simulink model "ScriptDemo"  (R2022b)
settings: configuration reference "TmVcThermal_Configuration_sub" (kept outside this file)
undefined symbols (not defined in the file or in its folder): aaaa, bbbb, cTmComprCtrl_D_u8HvacFlowTable_db, cTmComprCtrl_D_u8HvacFlowTable_sw, cTmComprCtrl_n_i16ChillCmpIMax, cTmComprCtrl_n_i16ChillCmpIMin, cTmComprCtrl_n_i16ChillCmpIMin666, cTmComprCtrl_n_i16ChillCmpPMax, cTmComprCtrl_n_i16ChillCmpPMin, cTmComprCtrl_n_i16CmpChillCoolRpmKiMax, cTmComprCtrl_n_i16CmpChillCoolRpmKiMin, cTmComprCtrl_n_i16CmpChillCoolRpmKpMax, cTmComprCtrl_n_i16CmpChillCoolRpmKpMin, cTmComprCtrl_n_i16CmpCoolRpmKiMax, cTmComprCtrl_n_i16CmpCoolRpmKiMin, cTmComprCtrl_n_i16CmpCoolRpmKpMax, cTmComprCtrl_n_i16CmpCoolRpmKpMin, cTmComprCtrl_n_i16SM4CmpHeatKiMax, cTmComprCtrl_n_i16SM4CmpHeatKiMin, cTmComprCtrl_n_i16SM4CmpHeatKpMax, cTmComprCtrl_n_i16SM4CmpHeatKpMin, cTmComprCtrl_n_i16SM5CmpHeatKiMax, cTmComprCtrl_n_i16SM5CmpHeatKiMin, cTmComprCtrl_n_i16SM5CmpHeatKpMax, cTmComprCtrl_n_i16SM5CmpHeatKpMin, cTmComprCtrl_n_i16SM6CmpHeatKiMax, cTmComprCtrl_n_i16SM6CmpHeatKiMin, cTmComprCtrl_n_i16SM6CmpHeatKpMax, cTmComprCtrl_n_i16SM6CmpHeatKpMin, cTmComprCtrl_n_u16CmpMaxSpdFanFltLimt, cTmComprCtrl_n_u16CmpMaxSpdLoSidePFltLimt, cTmComprCtrl_n_u16CmpMaxSpdSensorFltLimt, cTmComprCtrl_n_u16CompMinRpm, cTmComprCtrl_n_u16CompRpmIncThres, cTmComprCtrl_t_u16BattCooltFFPeriod, cTmComprCtrl_t_u16BattCooltPIPeriod, cTmComprCtrl_t_u16CmpCoolFFPeriod, cTmComprCtrl_t_u16CmpCoolPIPeriod, cTmComprCtrl_t_u16CoolCmpChillFFPeriod, cTmComprCtrl_t_u16CoolCmpChillPIPeriod, cTmComprCtrl_t_u16SM4CmpHeatFFPeriod, cTmComprCtrl_t_u16SM4CmpHeatPIPeriod, cTmComprCtrl_t_u16SM5CmpHeatFFPeriod, cTmComprCtrl_t_u16SM5CmpHeatPIPeriod, cTmComprCtrl_t_u16SM6CmpHeatFFPeriod, cTmComprCtrl_t_u16SM6CmpHeatPIPeriod, cTmComprCtrl_Te_EvapClearInteg, cTmComprCtrl_Te_i16HpReqTempSaturoffset, cTmComprCtrl_Te_i16SatLpReplaceDiff, cTmComprCtrl_Te_i16SM3BatDiffStartEvapDecOffset, cTmComprCtrl_Te_i16SM3EvapLo, cTmComprCtrl_Te_i16SM3TBatDiffEntEvapDecOffset, cTmComprCtrl_Te_i16SM3TBatDiffEntEvapDecOffsetQuit, cTmComprCtrl_Te_s32ErrCmpChillPIContinueCoolH, cTmComprCtrl_Te_s32ErrCmpChillPIContinueCoolL, cTmComprCtrl_Te_s32ErrCmpPIContinueChillH, cTmComprCtrl_Te_s32ErrCmpPIContinueChillL, cTmComprCtrl_Te_s32ErrCmpPIContinueCoolH, cTmComprCtrl_Te_s32ErrCmpPIContinueCoolL, cTmComprCtrl_Te_s32ErrCmpPIContinueHeatH ... (+398)
libraries: simulink x846, PCMULib x711, simulink_need_slupdate x4
(part 25 of 49)

== system ScriptDemo/Create/createSigOnLine/Before2/Before ==
  note: % 目的: 为输出端口创建debug 及对应的输入模块
      | [cnt] = createDebug(gcs)
  sTmRefriVlvCtrl_X_s32CEXVPosReqIn : Inport  OutDataTypeStr=single
  sTmRefriVlvCtrl_X_s32EEXVPosReqIn : Inport  Port=2  OutDataTypeStr=single
  sTmRefriVlvCtrl_X_s32BEXVPosReqIn : Inport  Port=3  OutDataTypeStr=single
  yTmRefriVlvCtrl_B_HpcCexvMovEnableIn : Inport  Port=4  OutDataTypeStr=boolean
  sTmRefriVlvCtrl_Z_u8CEXVInitStateIn : Inport  Port=5  OutDataTypeStr=uint8
  yTmRefriVlvCtrl_B_CexvCalibReqIn : Inport  Port=6  OutDataTypeStr=boolean
  yTmRefriVlvCtrl_B_HpcEexvMovEnableIn : Inport  Port=7  OutDataTypeStr=boolean
  sTmRefriVlvCtrl_Z_u8EEXVInitStateIn : Inport  Port=8  OutDataTypeStr=uint8
  yTmRefriVlvCtrl_B_EexvCalibReqIn : Inport  Port=9  OutDataTypeStr=boolean
  yTmRefriVlvCtrl_B_HpcBexvMovEnableIn : Inport  Port=10  OutDataTypeStr=boolean
  sTmRefriVlvCtrl_Z_u8BEXVInitStateIn : Inport  Port=11  OutDataTypeStr=uint8
  yTmRefriVlvCtrl_B_BexvCalibReqIn : Inport  Port=12  OutDataTypeStr=boolean
  sTmRefriVlvCtrl_X_s32SM3BexvMaxPosIn : Inport  Port=13  OutDataTypeStr=single
  yTmRefriVlvCtrl_B_EvapBattTLimBexvEnaIn : Inport  Port=14  OutDataTypeStr=boolean
  sTmRefriVlvCtrl_D_u8EexvRefriSwitchStIn : Inport  Port=15  OutDataTypeStr=uint8
  sTmRefriVlvCtrl_D_u8CexvRefriSwitchStIn : Inport  Port=16  OutDataTypeStr=uint8
  sTmRefriVlvCtrl_D_u8BexvRefriSwitchStIn : Inport  Port=17  OutDataTypeStr=uint8
  OutDebug : PCMULib/Interface/OutdebugRvs  SWI=cTmRefriVlvCtrl_X_s32CEXVPosReq_sw  DBI=cTmRefriVlvCtrl_X_s32CEXVPosReq_db
      settings: SourceProductName=PCMULib
  OutDebug1 : PCMULib/Interface/OutdebugRvs  SWI=cTmRefriVlvCtrl_X_s32EEXVPosReq_sw  DBI=cTmRefriVlvCtrl_X_s32EEXVPosReq_db
      settings: SourceProductName=PCMULib
  OutDebug10 : PCMULib/Interface/OutdebugRvs  SWI=cTmRefriVlvCtrl_Z_u8BEXVInitState_sw  DBI=cTmRefriVlvCtrl_Z_u8BEXVInitState_db
      settings: SourceProductName=PCMULib
  OutDebug11 : PCMULib/Interface/OutdebugRvs  SWI=cTmRefriVlvCtrl_B_BexvCalibReq_sw  DBI=cTmRefriVlvCtrl_B_BexvCalibReq_db
      settings: SourceProductName=PCMULib
  OutDebug12 : PCMULib/Interface/OutdebugRvs  SWI=cTmRefriVlvCtrl_X_s32SM3BexvMaxPos_sw  DBI=cTmRefriVlvCtrl_X_s32SM3BexvMaxPos_db
      settings: SourceProductName=PCMULib
  OutDebug13 : PCMULib/Interface/OutdebugRvs  SWI=cTmRefriVlvCtrl_B_EvapBattTLimBexvEna_sw  DBI=cTmRefriVlvCtrl_B_EvapBattTLimBexvEna_db
      settings: SourceProductName=PCMULib
  OutDebug14 : PCMULib/Interface/OutdebugRvs  SWI=cTmRefriVlvCtrl_D_u8EexvRefriSwitchSt_sw  DBI=cTmRefriVlvCtrl_D_u8EexvRefriSwitchSt_db
      settings: SourceProductName=PCMULib
  OutDebug15 : PCMULib/Interface/OutdebugRvs  SWI=cTmRefriVlvCtrl_D_u8CexvRefriSwitchSt_sw  DBI=cTmRefriVlvCtrl_D_u8CexvRefriSwitchSt_db
      settings: SourceProductName=PCMULib
  OutDebug16 : PCMULib/Interface/OutdebugRvs  SWI=cTmRefriVlvCtrl_D_u8BexvRefriSwitchSt_sw  DBI=cTmRefriVlvCtrl_D_u8BexvRefriSwitchSt_db
      settings: SourceProductName=PCMULib
  OutDebug2 : PCMULib/Interface/OutdebugRvs  SWI=cTmRefriVlvCtrl_X_s32BEXVPosReq_sw  DBI=cTmRefriVlvCtrl_X_s32BEXVPosReq_db
      settings: SourceProductName=PCMULib
  OutDebug3 : PCMULib/Interface/OutdebugRvs  SWI=cTmRefriVlvCtrl_B_HpcCexvMovEnable_sw  DBI=cTmRefriVlvCtrl_B_HpcCexvMovEnable_db
      settings: SourceProductName=PCMULib
  OutDebug4 : PCMULib/Interface/OutdebugRvs  SWI=cTmRefriVlvCtrl_Z_u8CEXVInitState_sw  DBI=cTmRefriVlvCtrl_Z_u8CEXVInitState_db
      settings: SourceProductName=PCMULib
  OutDebug5 : PCMULib/Interface/OutdebugRvs  SWI=cTmRefriVlvCtrl_B_CexvCalibReq_sw  DBI=cTmRefriVlvCtrl_B_CexvCalibReq_db
      settings: SourceProductName=PCMULib
  OutDebug6 : PCMULib/Interface/OutdebugRvs  SWI=cTmRefriVlvCtrl_B_HpcEexvMovEnable_sw  DBI=cTmRefriVlvCtrl_B_HpcEexvMovEnable_db
      settings: SourceProductName=PCMULib
  OutDebug7 : PCMULib/Interface/OutdebugRvs  SWI=cTmRefriVlvCtrl_Z_u8EEXVInitState_sw  DBI=cTmRefriVlvCtrl_Z_u8EEXVInitState_db
      settings: SourceProductName=PCMULib
  OutDebug8 : PCMULib/Interface/OutdebugRvs  SWI=cTmRefriVlvCtrl_B_EexvCalibReq_sw  DBI=cTmRefriVlvCtrl_B_EexvCalibReq_db
      settings: SourceProductName=PCMULib
  OutDebug9 : PCMULib/Interface/OutdebugRvs  SWI=cTmRefriVlvCtrl_B_HpcBexvMovEnable_sw  DBI=cTmRefriVlvCtrl_B_HpcBexvMovEnable_db
      settings: SourceProductName=PCMULib
  sTmRefriVlvCtrl_X_s32CEXVPosReq : Outport  OutDataTypeStr=single
  sTmRefriVlvCtrl_X_s32EEXVPosReq : Outport  Port=2  OutDataTypeStr=single
  sTmRefriVlvCtrl_X_s32BEXVPosReq : Outport  Port=3  OutDataTypeStr=single
  yTmRefriVlvCtrl_B_HpcCexvMovEnable : Outport  Port=4  OutDataTypeStr=boolean
  sTmRefriVlvCtrl_Z_u8CEXVInitState : Outport  Port=5  OutDataTypeStr=uint8
  yTmRefriVlvCtrl_B_CexvCalibReq : Outport  Port=6  OutDataTypeStr=boolean
  yTmRefriVlvCtrl_B_HpcEexvMovEnable : Outport  Port=7  OutDataTypeStr=boolean
  sTmRefriVlvCtrl_Z_u8EEXVInitState : Outport  Port=8  OutDataTypeStr=uint8
  yTmRefriVlvCtrl_B_EexvCalibReq : Outport  Port=9  OutDataTypeStr=boolean
  yTmRefriVlvCtrl_B_HpcBexvMovEnable : Outport  Port=10  OutDataTypeStr=boolean
  sTmRefriVlvCtrl_Z_u8BEXVInitState : Outport  Port=11  OutDataTypeStr=uint8
  yTmRefriVlvCtrl_B_BexvCalibReq : Outport  Port=12  OutDataTypeStr=boolean
  sTmRefriVlvCtrl_X_s32SM3BexvMaxPos : Outport  Port=13  OutDataTypeStr=single
  yTmRefriVlvCtrl_B_EvapBattTLimBexvEna : Outport  Port=14  OutDataTypeStr=boolean
  sTmRefriVlvCtrl_D_u8EexvRefriSwitchSt : Outport  Port=15  OutDataTypeStr=uint8
  sTmRefriVlvCtrl_D_u8CexvRefriSwitchSt : Outport  Port=16  OutDataTypeStr=uint8
  sTmRefriVlvCtrl_D_u8BexvRefriSwitchSt : Outport  Port=17  OutDataTypeStr=uint8
  wires:
  sTmRefriVlvCtrl_X_s32SM3BexvMaxPosIn/1 -> OutDebug12/1
  OutDebug12/1 -> sTmRefriVlvCtrl_X_s32SM3BexvMaxPos/1
  sTmRefriVlvCtrl_X_s32BEXVPosReqIn/1 -> OutDebug2/1
  OutDebug2/1 -> sTmRefriVlvCtrl_X_s32BEXVPosReq/1
  OutDebug16/1 -> sTmRefriVlvCtrl_D_u8BexvRefriSwitchSt/1
  sTmRefriVlvCtrl_D_u8EexvRefriSwitchStIn/1 -> OutDebug14/1
  OutDebug5/1 -> yTmRefriVlvCtrl_B_CexvCalibReq/1
  OutDebug3/1 -> yTmRefriVlvCtrl_B_HpcCexvMovEnable/1
  sTmRefriVlvCtrl_Z_u8CEXVInitStateIn/1 -> OutDebug4/1
  OutDebug4/1 -> sTmRefriVlvCtrl_Z_u8CEXVInitState/1
  sTmRefriVlvCtrl_D_u8BexvRefriSwitchStIn/1 -> OutDebug16/1
  OutDebug1/1 -> sTmRefriVlvCtrl_X_s32EEXVPosReq/1
  OutDebug14/1 -> sTmRefriVlvCtrl_D_u8EexvRefriSwitchSt/1
  yTmRefriVlvCtrl_B_CexvCalibReqIn/1 -> OutDebug5/1
  sTmRefriVlvCtrl_X_s32EEXVPosReqIn/1 -> OutDebug1/1
  yTmRefriVlvCtrl_B_HpcCexvMovEnableIn/1 -> OutDebug3/1
  yTmRefriVlvCtrl_B_EvapBattTLimBexvEnaIn/1 -> OutDebug13/1
  OutDebug13/1 -> yTmRefriVlvCtrl_B_EvapBattTLimBexvEna/1
  sTmRefriVlvCtrl_Z_u8BEXVInitStateIn/1 -> OutDebug10/1
  OutDebug10/1 -> sTmRefriVlvCtrl_Z_u8BEXVInitState/1
  sTmRefriVlvCtrl_D_u8CexvRefriSwitchStIn/1 -> OutDebug15/1
  OutDebug15/1 -> sTmRefriVlvCtrl_D_u8CexvRefriSwitchSt/1
  OutDebug/1 -> sTmRefriVlvCtrl_X_s32CEXVPosReq/1
  OutDebug7/1 -> sTmRefriVlvCtrl_Z_u8EEXVInitState/1
  OutDebug8/1 -> yTmRefriVlvCtrl_B_EexvCalibReq/1
  yTmRefriVlvCtrl_B_EexvCalibReqIn/1 -> OutDebug8/1
  sTmRefriVlvCtrl_X_s32CEXVPosReqIn/1 -> OutDebug/1
  OutDebug6/1 -> yTmRefriVlvCtrl_B_HpcEexvMovEnable/1
  yTmRefriVlvCtrl_B_HpcEexvMovEnableIn/1 -> OutDebug6/1
  sTmRefriVlvCtrl_Z_u8EEXVInitStateIn/1 -> OutDebug7/1
  yTmRefriVlvCtrl_B_HpcBexvMovEnableIn/1 -> OutDebug9/1
  OutDebug9/1 -> yTmRefriVlvCtrl_B_HpcBexvMovEnable/1
  yTmRefriVlvCtrl_B_BexvCalibReqIn/1 -> OutDebug11/1
  OutDebug11/1 -> yTmRefriVlvCtrl_B_BexvCalibReq/1

== system ScriptDemo/Create/createSigOnLine/Before3/Before ==
  note: % 目的: 为输出端口创建debug 及对应的输入模块
      | [cnt] = createDebug(gcs)
  sTmRefriVlvCtrl_X_s32CEXVPosReqIn : Inport  OutDataTypeStr=single
  sTmRefriVlvCtrl_X_s32EEXVPosReqIn : Inport  Port=2  OutDataTypeStr=single
  sTmRefriVlvCtrl_X_s32BEXVPosReqIn : Inport  Port=3  OutDataTypeStr=single
  yTmRefriVlvCtrl_B_HpcCexvMovEnableIn : Inport  Port=4  OutDataTypeStr=boolean
  sTmRefriVlvCtrl_Z_u8CEXVInitStateIn : Inport  Port=5  OutDataTypeStr=uint8
  yTmRefriVlvCtrl_B_CexvCalibReqIn : Inport  Port=6  OutDataTypeStr=boolean
  yTmRefriVlvCtrl_B_HpcEexvMovEnableIn : Inport  Port=7  OutDataTypeStr=boolean
  sTmRefriVlvCtrl_Z_u8EEXVInitStateIn : Inport  Port=8  OutDataTypeStr=uint8
  yTmRefriVlvCtrl_B_EexvCalibReqIn : Inport  Port=9  OutDataTypeStr=boolean
  yTmRefriVlvCtrl_B_HpcBexvMovEnableIn : Inport  Port=10  OutDataTypeStr=boolean
  sTmRefriVlvCtrl_Z_u8BEXVInitStateIn : Inport  Port=11  OutDataTypeStr=uint8
  yTmRefriVlvCtrl_B_BexvCalibReqIn : Inport  Port=12  OutDataTypeStr=boolean
  sTmRefriVlvCtrl_X_s32SM3BexvMaxPosIn : Inport  Port=13  OutDataTypeStr=single
  yTmRefriVlvCtrl_B_EvapBattTLimBexvEnaIn : Inport  Port=14  OutDataTypeStr=boolean
  sTmRefriVlvCtrl_D_u8EexvRefriSwitchStIn : Inport  Port=15  OutDataTypeStr=uint8
  sTmRefriVlvCtrl_D_u8CexvRefriSwitchStIn : Inport  Port=16  OutDataTypeStr=uint8
  sTmRefriVlvCtrl_D_u8BexvRefriSwitchStIn : Inport  Port=17  OutDataTypeStr=uint8
  OutDebug : PCMULib/Interface/OutdebugRvs  SWI=cTmRefriVlvCtrl_X_s32CEXVPosReq_sw  DBI=cTmRefriVlvCtrl_X_s32CEXVPosReq_db
      settings: SourceProductName=PCMULib
  OutDebug1 : PCMULib/Interface/OutdebugRvs  SWI=cTmRefriVlvCtrl_X_s32EEXVPosReq_sw  DBI=cTmRefriVlvCtrl_X_s32EEXVPosReq_db
      settings: SourceProductName=PCMULib
  OutDebug10 : PCMULib/Interface/OutdebugRvs  SWI=cTmRefriVlvCtrl_Z_u8BEXVInitState_sw  DBI=cTmRefriVlvCtrl_Z_u8BEXVInitState_db
      settings: SourceProductName=PCMULib
  OutDebug11 : PCMULib/Interface/OutdebugRvs  SWI=cTmRefriVlvCtrl_B_BexvCalibReq_sw  DBI=cTmRefriVlvCtrl_B_BexvCalibReq_db
      settings: SourceProductName=PCMULib
  OutDebug12 : PCMULib/Interface/OutdebugRvs  SWI=cTmRefriVlvCtrl_X_s32SM3BexvMaxPos_sw  DBI=cTmRefriVlvCtrl_X_s32SM3BexvMaxPos_db
      settings: SourceProductName=PCMULib
  OutDebug13 : PCMULib/Interface/OutdebugRvs  SWI=cTmRefriVlvCtrl_B_EvapBattTLimBexvEna_sw  DBI=cTmRefriVlvCtrl_B_EvapBattTLimBexvEna_db
      settings: SourceProductName=PCMULib
  OutDebug14 : PCMULib/Interface/OutdebugRvs  SWI=cTmRefriVlvCtrl_D_u8EexvRefriSwitchSt_sw  DBI=cTmRefriVlvCtrl_D_u8EexvRefriSwitchSt_db
      settings: SourceProductName=PCMULib
  OutDebug15 : PCMULib/Interface/OutdebugRvs  SWI=cTmRefriVlvCtrl_D_u8CexvRefriSwitchSt_sw  DBI=cTmRefriVlvCtrl_D_u8CexvRefriSwitchSt_db
      settings: SourceProductName=PCMULib
  OutDebug16 : PCMULib/Interface/OutdebugRvs  SWI=cTmRefriVlvCtrl_D_u8BexvRefriSwitchSt_sw  DBI=cTmRefriVlvCtrl_D_u8BexvRefriSwitchSt_db
      settings: SourceProductName=PCMULib
  OutDebug2 : PCMULib/Interface/OutdebugRvs  SWI=cTmRefriVlvCtrl_X_s32BEXVPosReq_sw  DBI=cTmRefriVlvCtrl_X_s32BEXVPosReq_db
      settings: SourceProductName=PCMULib
  OutDebug3 : PCMULib/Interface/OutdebugRvs  SWI=cTmRefriVlvCtrl_B_HpcCexvMovEnable_sw  DBI=cTmRefriVlvCtrl_B_HpcCexvMovEnable_db
      settings: SourceProductName=PCMULib
  OutDebug4 : PCMULib/Interface/OutdebugRvs  SWI=cTmRefriVlvCtrl_Z_u8CEXVInitState_sw  DBI=cTmRefriVlvCtrl_Z_u8CEXVInitState_db
      settings: SourceProductName=PCMULib
  OutDebug5 : PCMULib/Interface/OutdebugRvs  SWI=cTmRefriVlvCtrl_B_CexvCalibReq_sw  DBI=cTmRefriVlvCtrl_B_CexvCalibReq_db
      settings: SourceProductName=PCMULib
  OutDebug6 : PCMULib/Interface/OutdebugRvs  SWI=cTmRefriVlvCtrl_B_HpcEexvMovEnable_sw  DBI=cTmRefriVlvCtrl_B_HpcEexvMovEnable_db
      settings: SourceProductName=PCMULib
  OutDebug7 : PCMULib/Interface/OutdebugRvs  SWI=cTmRefriVlvCtrl_Z_u8EEXVInitState_sw  DBI=cTmRefriVlvCtrl_Z_u8EEXVInitState_db
      settings: SourceProductName=PCMULib
  OutDebug8 : PCMULib/Interface/OutdebugRvs  SWI=cTmRefriVlvCtrl_B_EexvCalibReq_sw  DBI=cTmRefriVlvCtrl_B_EexvCalibReq_db
      settings: SourceProductName=PCMULib
  OutDebug9 : PCMULib/Interface/OutdebugRvs  SWI=cTmRefriVlvCtrl_B_HpcBexvMovEnable_sw  DBI=cTmRefriVlvCtrl_B_HpcBexvMovEnable_db
      settings: SourceProductName=PCMULib
  sTmRefriVlvCtrl_X_s32CEXVPosReq : Outport  OutDataTypeStr=single
  sTmRefriVlvCtrl_X_s32EEXVPosReq : Outport  Port=2  OutDataTypeStr=single
  sTmRefriVlvCtrl_X_s32BEXVPosReq : Outport  Port=3  OutDataTypeStr=single
  yTmRefriVlvCtrl_B_HpcCexvMovEnable : Outport  Port=4  OutDataTypeStr=boolean
  sTmRefriVlvCtrl_Z_u8CEXVInitState : Outport  Port=5  OutDataTypeStr=uint8
  yTmRefriVlvCtrl_B_CexvCalibReq : Outport  Port=6  OutDataTypeStr=boolean
  yTmRefriVlvCtrl_B_HpcEexvMovEnable : Outport  Port=7  OutDataTypeStr=boolean
  sTmRefriVlvCtrl_Z_u8EEXVInitState : Outport  Port=8  OutDataTypeStr=uint8
  yTmRefriVlvCtrl_B_EexvCalibReq : Outport  Port=9  OutDataTypeStr=boolean
  yTmRefriVlvCtrl_B_HpcBexvMovEnable : Outport  Port=10  OutDataTypeStr=boolean
  sTmRefriVlvCtrl_Z_u8BEXVInitState : Outport  Port=11  OutDataTypeStr=uint8
  yTmRefriVlvCtrl_B_BexvCalibReq : Outport  Port=12  OutDataTypeStr=boolean
  sTmRefriVlvCtrl_X_s32SM3BexvMaxPos : Outport  Port=13  OutDataTypeStr=single
  yTmRefriVlvCtrl_B_EvapBattTLimBexvEna : Outport  Port=14  OutDataTypeStr=boolean
  sTmRefriVlvCtrl_D_u8EexvRefriSwitchSt : Outport  Port=15  OutDataTypeStr=uint8
  sTmRefriVlvCtrl_D_u8CexvRefriSwitchSt : Outport  Port=16  OutDataTypeStr=uint8
  sTmRefriVlvCtrl_D_u8BexvRefriSwitchSt : Outport  Port=17  OutDataTypeStr=uint8
  wires:
  sTmRefriVlvCtrl_X_s32SM3BexvMaxPosIn/1 -> OutDebug12/1
  OutDebug12/1 -> sTmRefriVlvCtrl_X_s32SM3BexvMaxPos/1
  sTmRefriVlvCtrl_X_s32BEXVPosReqIn/1 -> OutDebug2/1
  OutDebug2/1 -> sTmRefriVlvCtrl_X_s32BEXVPosReq/1
  OutDebug16/1 -> sTmRefriVlvCtrl_D_u8BexvRefriSwitchSt/1
  sTmRefriVlvCtrl_D_u8EexvRefriSwitchStIn/1 -> OutDebug14/1
  OutDebug5/1 -> yTmRefriVlvCtrl_B_CexvCalibReq/1
  OutDebug3/1 -> yTmRefriVlvCtrl_B_HpcCexvMovEnable/1
  sTmRefriVlvCtrl_Z_u8CEXVInitStateIn/1 -> OutDebug4/1
  OutDebug4/1 -> sTmRefriVlvCtrl_Z_u8CEXVInitState/1
  sTmRefriVlvCtrl_D_u8BexvRefriSwitchStIn/1 -> OutDebug16/1
  OutDebug1/1 -> sTmRefriVlvCtrl_X_s32EEXVPosReq/1
  OutDebug14/1 -> sTmRefriVlvCtrl_D_u8EexvRefriSwitchSt/1
  yTmRefriVlvCtrl_B_CexvCalibReqIn/1 -> OutDebug5/1
  sTmRefriVlvCtrl_X_s32EEXVPosReqIn/1 -> OutDebug1/1
  yTmRefriVlvCtrl_B_HpcCexvMovEnableIn/1 -> OutDebug3/1
  yTmRefriVlvCtrl_B_EvapBattTLimBexvEnaIn/1 -> OutDebug13/1
  OutDebug13/1 -> yTmRefriVlvCtrl_B_EvapBattTLimBexvEna/1
  sTmRefriVlvCtrl_Z_u8BEXVInitStateIn/1 -> OutDebug10/1
  OutDebug10/1 -> sTmRefriVlvCtrl_Z_u8BEXVInitState/1
  sTmRefriVlvCtrl_D_u8CexvRefriSwitchStIn/1 -> OutDebug15/1
  OutDebug15/1 -> sTmRefriVlvCtrl_D_u8CexvRefriSwitchSt/1
  OutDebug/1 -> sTmRefriVlvCtrl_X_s32CEXVPosReq/1
  OutDebug7/1 -> sTmRefriVlvCtrl_Z_u8EEXVInitState/1
  OutDebug8/1 -> yTmRefriVlvCtrl_B_EexvCalibReq/1
  yTmRefriVlvCtrl_B_EexvCalibReqIn/1 -> OutDebug8/1
  sTmRefriVlvCtrl_X_s32CEXVPosReqIn/1 -> OutDebug/1
  OutDebug6/1 -> yTmRefriVlvCtrl_B_HpcEexvMovEnable/1
  yTmRefriVlvCtrl_B_HpcEexvMovEnableIn/1 -> OutDebug6/1
  sTmRefriVlvCtrl_Z_u8EEXVInitStateIn/1 -> OutDebug7/1
  yTmRefriVlvCtrl_B_HpcBexvMovEnableIn/1 -> OutDebug9/1
  OutDebug9/1 -> yTmRefriVlvCtrl_B_HpcBexvMovEnable/1
  yTmRefriVlvCtrl_B_BexvCalibReqIn/1 -> OutDebug11/1
  OutDebug11/1 -> yTmRefriVlvCtrl_B_BexvCalibReq/1

== system ScriptDemo/Create/createSigOnLine/Before4/Before ==
  note: % 目的: 为输出端口创建debug 及对应的输入模块
      | [cnt] = createDebug(gcs)
  sTmRefriVlvCtrl_X_s32CEXVPosReqIn : Inport  OutDataTypeStr=single
  sTmRefriVlvCtrl_X_s32EEXVPosReqIn : Inport  Port=2  OutDataTypeStr=single
  sTmRefriVlvCtrl_X_s32BEXVPosReqIn : Inport  Port=3  OutDataTypeStr=single
  yTmRefriVlvCtrl_B_HpcCexvMovEnableIn : Inport  Port=4  OutDataTypeStr=boolean
  sTmRefriVlvCtrl_Z_u8CEXVInitStateIn : Inport  Port=5  OutDataTypeStr=uint8
  yTmRefriVlvCtrl_B_CexvCalibReqIn : Inport  Port=6  OutDataTypeStr=boolean
  yTmRefriVlvCtrl_B_HpcEexvMovEnableIn : Inport  Port=7  OutDataTypeStr=boolean
  sTmRefriVlvCtrl_Z_u8EEXVInitStateIn : Inport  Port=8  OutDataTypeStr=uint8
  yTmRefriVlvCtrl_B_EexvCalibReqIn : Inport  Port=9  OutDataTypeStr=boolean
  yTmRefriVlvCtrl_B_HpcBexvMovEnableIn : Inport  Port=10  OutDataTypeStr=boolean
  sTmRefriVlvCtrl_Z_u8BEXVInitStateIn : Inport  Port=11  OutDataTypeStr=uint8
  yTmRefriVlvCtrl_B_BexvCalibReqIn : Inport  Port=12  OutDataTypeStr=boolean
  sTmRefriVlvCtrl_X_s32SM3BexvMaxPosIn : Inport  Port=13  OutDataTypeStr=single
  yTmRefriVlvCtrl_B_EvapBattTLimBexvEnaIn : Inport  Port=14  OutDataTypeStr=boolean
  sTmRefriVlvCtrl_D_u8EexvRefriSwitchStIn : Inport  Port=15  OutDataTypeStr=uint8
  sTmRefriVlvCtrl_D_u8CexvRefriSwitchStIn : Inport  Port=16  OutDataTypeStr=uint8
  sTmRefriVlvCtrl_D_u8BexvRefriSwitchStIn : Inport  Port=17  OutDataTypeStr=uint8
  OutDebug : PCMULib/Interface/OutdebugRvs  SWI=cTmRefriVlvCtrl_X_s32CEXVPosReq_sw  DBI=cTmRefriVlvCtrl_X_s32CEXVPosReq_db
      settings: SourceProductName=PCMULib
  OutDebug1 : PCMULib/Interface/OutdebugRvs  SWI=cTmRefriVlvCtrl_X_s32EEXVPosReq_sw  DBI=cTmRefriVlvCtrl_X_s32EEXVPosReq_db
      settings: SourceProductName=PCMULib
  OutDebug10 : PCMULib/Interface/OutdebugRvs  SWI=cTmRefriVlvCtrl_Z_u8BEXVInitState_sw  DBI=cTmRefriVlvCtrl_Z_u8BEXVInitState_db
      settings: SourceProductName=PCMULib
  OutDebug11 : PCMULib/Interface/OutdebugRvs  SWI=cTmRefriVlvCtrl_B_BexvCalibReq_sw  DBI=cTmRefriVlvCtrl_B_BexvCalibReq_db
      settings: SourceProductName=PCMULib
  OutDebug12 : PCMULib/Interface/OutdebugRvs  SWI=cTmRefriVlvCtrl_X_s32SM3BexvMaxPos_sw  DBI=cTmRefriVlvCtrl_X_s32SM3BexvMaxPos_db
      settings: SourceProductName=PCMULib
  OutDebug13 : PCMULib/Interface/OutdebugRvs  SWI=cTmRefriVlvCtrl_B_EvapBattTLimBexvEna_sw  DBI=cTmRefriVlvCtrl_B_EvapBattTLimBexvEna_db
      settings: SourceProductName=PCMULib
  OutDebug14 : PCMULib/Interface/OutdebugRvs  SWI=cTmRefriVlvCtrl_D_u8EexvRefriSwitchSt_sw  DBI=cTmRefriVlvCtrl_D_u8EexvRefriSwitchSt_db
      settings: SourceProductName=PCMULib
  OutDebug15 : PCMULib/Interface/OutdebugRvs  SWI=cTmRefriVlvCtrl_D_u8CexvRefriSwitchSt_sw  DBI=cTmRefriVlvCtrl_D_u8CexvRefriSwitchSt_db
      settings: SourceProductName=PCMULib
  OutDebug16 : PCMULib/Interface/OutdebugRvs  SWI=cTmRefriVlvCtrl_D_u8BexvRefriSwitchSt_sw  DBI=cTmRefriVlvCtrl_D_u8BexvRefriSwitchSt_db
      settings: SourceProductName=PCMULib
  OutDebug2 : PCMULib/Interface/OutdebugRvs  SWI=cTmRefriVlvCtrl_X_s32BEXVPosReq_sw  DBI=cTmRefriVlvCtrl_X_s32BEXVPosReq_db
      settings: SourceProductName=PCMULib
  OutDebug3 : PCMULib/Interface/OutdebugRvs  SWI=cTmRefriVlvCtrl_B_HpcCexvMovEnable_sw  DBI=cTmRefriVlvCtrl_B_HpcCexvMovEnable_db
      settings: SourceProductName=PCMULib
  OutDebug4 : PCMULib/Interface/OutdebugRvs  SWI=cTmRefriVlvCtrl_Z_u8CEXVInitState_sw  DBI=cTmRefriVlvCtrl_Z_u8CEXVInitState_db
      settings: SourceProductName=PCMULib
  OutDebug5 : PCMULib/Interface/OutdebugRvs  SWI=cTmRefriVlvCtrl_B_CexvCalibReq_sw  DBI=cTmRefriVlvCtrl_B_CexvCalibReq_db
      settings: SourceProductName=PCMULib
  OutDebug6 : PCMULib/Interface/OutdebugRvs  SWI=cTmRefriVlvCtrl_B_HpcEexvMovEnable_sw  DBI=cTmRefriVlvCtrl_B_HpcEexvMovEnable_db
      settings: SourceProductName=PCMULib
  OutDebug7 : PCMULib/Interface/OutdebugRvs  SWI=cTmRefriVlvCtrl_Z_u8EEXVInitState_sw  DBI=cTmRefriVlvCtrl_Z_u8EEXVInitState_db
      settings: SourceProductName=PCMULib
  OutDebug8 : PCMULib/Interface/OutdebugRvs  SWI=cTmRefriVlvCtrl_B_EexvCalibReq_sw  DBI=cTmRefriVlvCtrl_B_EexvCalibReq_db
      settings: SourceProductName=PCMULib
  OutDebug9 : PCMULib/Interface/OutdebugRvs  SWI=cTmRefriVlvCtrl_B_HpcBexvMovEnable_sw  DBI=cTmRefriVlvCtrl_B_HpcBexvMovEnable_db
      settings: SourceProductName=PCMULib
  sTmRefriVlvCtrl_X_s32CEXVPosReq : Outport  OutDataTypeStr=single
  sTmRefriVlvCtrl_X_s32EEXVPosReq : Outport  Port=2  OutDataTypeStr=single
  sTmRefriVlvCtrl_X_s32BEXVPosReq : Outport  Port=3  OutDataTypeStr=single
  yTmRefriVlvCtrl_B_HpcCexvMovEnable : Outport  Port=4  OutDataTypeStr=boolean
  sTmRefriVlvCtrl_Z_u8CEXVInitState : Outport  Port=5  OutDataTypeStr=uint8
  yTmRefriVlvCtrl_B_CexvCalibReq : Outport  Port=6  OutDataTypeStr=boolean
  yTmRefriVlvCtrl_B_HpcEexvMovEnable : Outport  Port=7  OutDataTypeStr=boolean
  sTmRefriVlvCtrl_Z_u8EEXVInitState : Outport  Port=8  OutDataTypeStr=uint8
  yTmRefriVlvCtrl_B_EexvCalibReq : Outport  Port=9  OutDataTypeStr=boolean
  yTmRefriVlvCtrl_B_HpcBexvMovEnable : Outport  Port=10  OutDataTypeStr=boolean
  sTmRefriVlvCtrl_Z_u8BEXVInitState : Outport  Port=11  OutDataTypeStr=uint8
  yTmRefriVlvCtrl_B_BexvCalibReq : Outport  Port=12  OutDataTypeStr=boolean
  sTmRefriVlvCtrl_X_s32SM3BexvMaxPos : Outport  Port=13  OutDataTypeStr=single
  yTmRefriVlvCtrl_B_EvapBattTLimBexvEna : Outport  Port=14  OutDataTypeStr=boolean
  sTmRefriVlvCtrl_D_u8EexvRefriSwitchSt : Outport  Port=15  OutDataTypeStr=uint8
  sTmRefriVlvCtrl_D_u8CexvRefriSwitchSt : Outport  Port=16  OutDataTypeStr=uint8
  sTmRefriVlvCtrl_D_u8BexvRefriSwitchSt : Outport  Port=17  OutDataTypeStr=uint8
  wires:
  sTmRefriVlvCtrl_X_s32SM3BexvMaxPosIn/1 -> OutDebug12/1
  OutDebug12/1 -> sTmRefriVlvCtrl_X_s32SM3BexvMaxPos/1
  sTmRefriVlvCtrl_X_s32BEXVPosReqIn/1 -> OutDebug2/1
  OutDebug2/1 -> sTmRefriVlvCtrl_X_s32BEXVPosReq/1
  OutDebug16/1 -> sTmRefriVlvCtrl_D_u8BexvRefriSwitchSt/1
  sTmRefriVlvCtrl_D_u8EexvRefriSwitchStIn/1 -> OutDebug14/1
  OutDebug5/1 -> yTmRefriVlvCtrl_B_CexvCalibReq/1
  OutDebug3/1 -> yTmRefriVlvCtrl_B_HpcCexvMovEnable/1
  sTmRefriVlvCtrl_Z_u8CEXVInitStateIn/1 -> OutDebug4/1
  OutDebug4/1 -> sTmRefriVlvCtrl_Z_u8CEXVInitState/1
  sTmRefriVlvCtrl_D_u8BexvRefriSwitchStIn/1 -> OutDebug16/1
  OutDebug1/1 -> sTmRefriVlvCtrl_X_s32EEXVPosReq/1
  OutDebug14/1 -> sTmRefriVlvCtrl_D_u8EexvRefriSwitchSt/1
  yTmRefriVlvCtrl_B_CexvCalibReqIn/1 -> OutDebug5/1
  sTmRefriVlvCtrl_X_s32EEXVPosReqIn/1 -> OutDebug1/1
  yTmRefriVlvCtrl_B_HpcCexvMovEnableIn/1 -> OutDebug3/1
  yTmRefriVlvCtrl_B_EvapBattTLimBexvEnaIn/1 -> OutDebug13/1
  OutDebug13/1 -> yTmRefriVlvCtrl_B_EvapBattTLimBexvEna/1
  sTmRefriVlvCtrl_Z_u8BEXVInitStateIn/1 -> OutDebug10/1
  OutDebug10/1 -> sTmRefriVlvCtrl_Z_u8BEXVInitState/1
  sTmRefriVlvCtrl_D_u8CexvRefriSwitchStIn/1 -> OutDebug15/1
  OutDebug15/1 -> sTmRefriVlvCtrl_D_u8CexvRefriSwitchSt/1
  OutDebug/1 -> sTmRefriVlvCtrl_X_s32CEXVPosReq/1
  OutDebug7/1 -> sTmRefriVlvCtrl_Z_u8EEXVInitState/1
  OutDebug8/1 -> yTmRefriVlvCtrl_B_EexvCalibReq/1
  yTmRefriVlvCtrl_B_EexvCalibReqIn/1 -> OutDebug8/1
  sTmRefriVlvCtrl_X_s32CEXVPosReqIn/1 -> OutDebug/1
  OutDebug6/1 -> yTmRefriVlvCtrl_B_HpcEexvMovEnable/1
  yTmRefriVlvCtrl_B_HpcEexvMovEnableIn/1 -> OutDebug6/1
  sTmRefriVlvCtrl_Z_u8EEXVInitStateIn/1 -> OutDebug7/1
  yTmRefriVlvCtrl_B_HpcBexvMovEnableIn/1 -> OutDebug9/1
  OutDebug9/1 -> yTmRefriVlvCtrl_B_HpcBexvMovEnable/1
  yTmRefriVlvCtrl_B_BexvCalibReqIn/1 -> OutDebug11/1
  OutDebug11/1 -> yTmRefriVlvCtrl_B_BexvCalibReq/1

== system ScriptDemo/Create/createSubMod/After/Fun666666_Req26245_DemoSub1 ==

== system ScriptDemo/Create/createSubMod/After/Fun666666_Req26246_DemoSub2 ==

== system ScriptDemo/Create/createSubMod/After/Fun666666_Req26247_DemoSub3 ==

== system ScriptDemo/Create/createSubMod/After/Fun666666_Req26248_DemoSub4 ==

== system ScriptDemo/Create/createSubMod/After/Fun666666_Req26249_DemoSub5 ==

== system ScriptDemo/Create/createSubMod/After/Fun888888_Req26250_DemoSub6 ==

== system ScriptDemo/Create/createSubMod/After/Fun888888_Req26251_DemoSub7 ==

== system ScriptDemo/Create/createSubMod/After/Fun888888_Req26252_DemoSub8 ==

== system ScriptDemo/Create/createSubMod/After/Fun888888_Req26253_DemoSub9 ==

== system ScriptDemo/Create/createSubMod/After/Fun888888_Req26254_DemoSub10 ==

== system ScriptDemo/Create/createSubmodInfo/After/tableChoose ==
  note: 快充
  note: 非快充，超充
  note: 电池有主动制冷需求
  note: 电池非正常制冷
  note: 超充
  note: 电池有主动制冷需求
  sTmSigProces_D_u8BattThermReq : Inport
  sTmIn_D_u8DCChrgSt : Inport  Port=2
  tab1 : Inport  Port=3
  tab2 : Inport  Port=4
  tab3 : Inport  Port=5
  Compare To Constant : simulink/Logic and Bit Operations/Compare To Constant  relop===  const=2  OutDataTypeStr=boolean
  Compare To Constant1 : simulink/Logic and Bit Operations/Compare To Constant  relop===  const=12  OutDataTypeStr=boolean
  Compare To Constant2 : simulink/Logic and Bit Operations/Compare To Constant  relop===  const=5  OutDataTypeStr=boolean
  Switch2 : Switch  Criteria=u2 ~= 0  SaturateOnIntegerOverflow=off  InputSameDT=off
  Switch4 : Switch  Criteria=u2 ~= 0  SaturateOnIntegerOverflow=off  InputSameDT=off
  Switch5 : Switch  Criteria=u2 ~= 0  SaturateOnIntegerOverflow=off  InputSameDT=off
  电池无主动制冷需求 : Constant  Value=0  OutDataTypeStr=uint16
  out : Outport
  wires:
  Compare To Constant1/1 -> Switch5/2
  tab1/1 -> Switch5/3
  tab3/1 -> Switch5/1
  tab2/1 -> Switch4/1
  sTmIn_D_u8DCChrgSt/1 -> Compare To Constant/1, Compare To Constant1/1
  Switch5/1 -> Switch4/3
  sTmSigProces_D_u8BattThermReq/1 -> Compare To Constant2/1
  Compare To Constant2/1 -> Switch2/2
  电池无主动制冷需求/1 -> Switch2/3
  Switch2/1 -> out/1
  Switch4/1 -> Switch2/1
  Compare To Constant/1 -> Switch4/2

== system ScriptDemo/Create/createSubmodInfo/Before/tableChoose ==
  note: 快充
  note: 非快充，超充
  note: 电池有主动制冷需求
  note: 电池非正常制冷
  note: 超充
  note: 电池有主动制冷需求
  sTmSigProces_D_u8BattThermReq : Inport
  sTmIn_D_u8DCChrgSt : Inport  Port=2
  tab1 : Inport  Port=3
  tab2 : Inport  Port=4
  tab3 : Inport  Port=5
  Compare To Constant : simulink/Logic and Bit Operations/Compare To Constant  relop===  const=2  OutDataTypeStr=boolean
  Compare To Constant1 : simulink/Logic and Bit Operations/Compare To Constant  relop===  const=12  OutDataTypeStr=boolean
  Compare To Constant2 : simulink/Logic and Bit Operations/Compare To Constant  relop===  const=5  OutDataTypeStr=boolean
  Switch2 : Switch  Criteria=u2 ~= 0  SaturateOnIntegerOverflow=off  InputSameDT=off
  Switch4 : Switch  Criteria=u2 ~= 0  SaturateOnIntegerOverflow=off  InputSameDT=off
  Switch5 : Switch  Criteria=u2 ~= 0  SaturateOnIntegerOverflow=off  InputSameDT=off
  电池无主动制冷需求 : Constant  Value=0  OutDataTypeStr=uint16
  out : Outport
  wires:
  Compare To Constant1/1 -> Switch5/2
  tab1/1 -> Switch5/3
  tab3/1 -> Switch5/1
  tab2/1 -> Switch4/1
  sTmIn_D_u8DCChrgSt/1 -> Compare To Constant/1, Compare To Constant1/1
  Switch5/1 -> Switch4/3
  sTmSigProces_D_u8BattThermReq/1 -> Compare To Constant2/1
  Compare To Constant2/1 -> Switch2/2
  电池无主动制冷需求/1 -> Switch2/3
  Switch2/1 -> out/1
  Switch4/1 -> Switch2/1
  Compare To Constant/1 -> Switch4/2

== system ScriptDemo/Create/createSwitchCase/After/Default ==
  Action Port : ActionPort  ActionPortLabel=default:
  xDefault_B_ChangeFinished : Outport
  rDefault_n_u16CompRpmReq : Outport  Port=2

== system ScriptDemo/Create/createSwitchCase/After/HoldSwitch ==
  Action Port : ActionPort  ActionPortLabel=case [ 17 ]:
  xHoldSwitch_B_ChangeFinished : Outport
  rHoldSwitch_n_u16CompRpmReq : Outport  Port=2

== system ScriptDemo/Create/createSwitchCase/After/ReduceRpm ==
  Action Port : ActionPort  ActionPortLabel=case [ 8 9 10 11 12 13 18 19 ]:
  xReduceRpm_B_ChangeFinished : Outport
  rReduceRpm_n_u16CompRpmReq : Outport  Port=2

== system ScriptDemo/Create/createSwitchCase/After/Stop ==
  Action Port : ActionPort  ActionPortLabel=case [ 1 ]:
  xStop_B_ChangeFinished : Outport
  rStop_n_u16CompRpmReq : Outport  Port=2

== system ScriptDemo/Create/createSwitchCase/After/Test ==
  Action Port : ActionPort  ActionPortLabel=case [ 20 ]:
  xTest_B_ChangeFinished : Outport
  rTest_n_u16CompRpmReq : Outport  Port=2

== system ScriptDemo/Create/createSwitchCase/After/Test2 ==
  Action Port : ActionPort  ActionPortLabel=case [ 21 ]:
  xTest2_B_ChangeFinished : Outport
  rTest2_n_u16CompRpmReq : Outport  Port=2

== system ScriptDemo/Create/createSwitchCase/After/Test3 ==
  Action Port : ActionPort  ActionPortLabel=case [ 22 ]:
  xTest3_B_ChangeFinished : Outport
  rTest3_n_u16CompRpmReq : Outport  Port=2

== system ScriptDemo/Create/createSwitchCase/After/Test4 ==
  Action Port : ActionPort  ActionPortLabel=case [ 23 ]:
  xTest4_B_ChangeFinished : Outport
  rTest4_n_u16CompRpmReq : Outport  Port=2

== system ScriptDemo/createHarness/ID31659_OffCodeState/bk/Subsystem ==
  Enable : EnablePort
  Constant : Constant  Value=0  OutDataTypeStr=uint8
  sTmComprCtrl_D_u8AirCondCmpsrStats : Outport
  wires:
  Constant/1 -> sTmComprCtrl_D_u8AirCondCmpsrStats/1

== system ScriptDemo/createHarness/ID31659_OffCodeState/bk/Subsystem1 ==
  Enable : EnablePort
  Constant : Constant  OutDataTypeStr=uint8
  sTmComprCtrl_D_u8AirCondCmpsrStats : Outport
  wires:
  Constant/1 -> sTmComprCtrl_D_u8AirCondCmpsrStats/1

== system ScriptDemo/createHarness/ID31659_OffCodeState/bk/Subsystem2 ==
  Enable : EnablePort
  Constant : Constant  Value=2  OutDataTypeStr=uint8
  sTmComprCtrl_D_u8AirCondCmpsrStats : Outport
  wires:
  Constant/1 -> sTmComprCtrl_D_u8AirCondCmpsrStats/1

== system ScriptDemo/createHarness/ID31659_OffCodeState/bk/Subsystem3 ==
  Enable : EnablePort
  Constant : Constant  Value=3  OutDataTypeStr=uint8
  sTmComprCtrl_D_u8AirCondCmpsrStats : Outport
  wires:
  Constant/1 -> sTmComprCtrl_D_u8AirCondCmpsrStats/1

== system ScriptDemo/createHarness/ID31659_OffCodeState/bk/Subsystem4 ==
  Enable : EnablePort
  Constant : Constant  Value=4  OutDataTypeStr=uint8
  sTmComprCtrl_D_u8AirCondCmpsrStats : Outport
  wires:
  Constant/1 -> sTmComprCtrl_D_u8AirCondCmpsrStats/1

== system ScriptDemo/createHarness/ID31659_OffCodeState/bk/Subsystem5 ==
  Enable : EnablePort
  Constant : Constant  Value=5  OutDataTypeStr=uint8
  sTmComprCtrl_D_u8AirCondCmpsrStats : Outport
  wires:
  Constant/1 -> sTmComprCtrl_D_u8AirCondCmpsrStats/1

== system ScriptDemo/createHarness/ID31659_OffCodeState/bk/Subsystem6 ==
  Enable : EnablePort
  Constant : Constant  Value=6  OutDataTypeStr=uint8
  sTmComprCtrl_D_u8AirCondCmpsrStats : Outport
  wires:
  Constant/1 -> sTmComprCtrl_D_u8AirCondCmpsrStats/1

== system ScriptDemo/createHarness/ID31659_OffCodeState/bk/Subsystem7 ==
  Enable : EnablePort
  Constant : Constant  Value=7  OutDataTypeStr=uint8
  sTmComprCtrl_D_u8AirCondCmpsrStats : Outport
  wires:
  Constant/1 -> sTmComprCtrl_D_u8AirCondCmpsrStats/1

== system ScriptDemo/Create/Model/createModGotoAll/After/AFFaultLimit ==
  sTmDiag_D_u8FanFltSt : Inport  OutDataTypeStr=uint8
  Compare To Constant : simulink/Logic and Bit Operations/Compare To Constant  relop=~=  const=0  OutDataTypeStr=boolean
  Constant : Constant  Value=cTmComprCtrl_n_u16CmpMaxSpdFanFltLimt  OutDataTypeStr=uint16
  Constant1 : Constant  Value=8000  OutDataTypeStr=uint16
  Switch : Switch  Criteria=u2 ~= 0  SaturateOnIntegerOverflow=off  InputSameDT=off
  rTmComprCtrl_n_u16CompMaxRpmAfFlt : Outport  OutDataTypeStr=uint16
  xTmComprCtrl_B_CmpFanFltLimtFlag : Outport  Port=2  OutDataTypeStr=boolean
  wires:
  Constant/1 -> Switch/1
  Constant1/1 -> Switch/3
  Switch/1 -> [rTmComprCtrl_n_u16CompMaxRpmAfFlt]  "rTmComprCtrl_n_u16CompMaxRpmAfFlt"
  sTmDiag_D_u8FanFltSt/1 -> [sTmDiag_D_u8FanFltSt]
  [rTmComprCtrl_n_u16CompMaxRpmAfFlt] -> rTmComprCtrl_n_u16CompMaxRpmAfFlt/1
  [sTmDiag_D_u8FanFltSt] -> Compare To Constant/1
  Compare To Constant/1 -> [xTmComprCtrl_B_CmpFanFltLimtFlag]
  [xTmComprCtrl_B_CmpFanFltLimtFlag] -> xTmComprCtrl_B_CmpFanFltLimtFlag/1
  [xTmComprCtrl_B_CmpFanFltLimtFlag] -> Switch/2

== system ScriptDemo/Create/Model/createModGotoAll/After/LoSidePFltLimt ==
  sTmDiag_D_u8LoSidePFltSt : Inport  OutDataTypeStr=uint8
  sTmIn_D_u8HeatPump : Inport  Port=2  OutDataTypeStr=uint8
  Compare To Constant : simulink/Logic and Bit Operations/Compare To Constant  relop=~=  const=0  OutDataTypeStr=boolean
  Compare To Constant1 : simulink/Logic and Bit Operations/Compare To Constant  relop=>  const=30  OutDataTypeStr=boolean
  Compare To Constant4 : simulink/Logic and Bit Operations/Compare To Constant  relop===  const=2  OutDataTypeStr=boolean
  Constant : Constant  Value=cTmComprCtrl_n_u16CmpMaxSpdLoSidePFltLimt  OutDataTypeStr=uint16
  Constant1 : Constant  Value=8000  OutDataTypeStr=uint16
  Logical Operator : Logic  Inputs=3  AllPortsSameDT=off  OutDataTypeStr=boolean
  Switch : Switch  Criteria=u2 ~= 0  SaturateOnIntegerOverflow=off  InputSameDT=off
  rTmComprCtrl_n_u16CompMaxRpmLoSidePFlt : Outport  OutDataTypeStr=uint16
  xTmComprCtrl_B_CmpLoSidePFltLimtFlag : Outport  Port=2  OutDataTypeStr=boolean
  wires:
  [xTmComprCtrl_B_CmpLoSidePFltLimtFlag] -> Switch/2
  [sTmSigProces_Te_s32TAmb] -> Compare To Constant1/1
  Constant/1 -> Switch/1
  Logical Operator/1 -> [xTmComprCtrl_B_CmpLoSidePFltLimtFlag]
  Switch/1 -> [rTmComprCtrl_n_u16CompMaxRpmLoSidePFlt]  "rTmComprCtrl_n_u16CompMaxRpmLoSidePFlt"
  [sTmDiag_D_u8LoSidePFltSt] -> Compare To Constant/1
  Constant1/1 -> Switch/3
  sTmDiag_D_u8LoSidePFltSt/1 -> [sTmDiag_D_u8LoSidePFltSt]
  ? -> [sTmSigProces_Te_s32TAmb]
  [rTmComprCtrl_n_u16CompMaxRpmLoSidePFlt] -> rTmComprCtrl_n_u16CompMaxRpmLoSidePFlt/1
  [xTmComprCtrl_B_CmpLoSidePFltLimtFlag] -> xTmComprCtrl_B_CmpLoSidePFltLimtFlag/1
  [sTmIn_D_u8HeatPump] -> Compare To Constant4/1
  Compare To Constant/1 -> Logical Operator/2
  Compare To Constant1/1 -> Logical Operator/3
  Compare To Constant4/1 -> Logical Operator/1
  sTmIn_D_u8HeatPump/1 -> [sTmIn_D_u8HeatPump]

== system ScriptDemo/Create/Model/createModGotoAll/After/SensFaultLimit ==
  sTmDiag_D_u8CmprDischrgTFltSt : Inport  OutDataTypeStr=uint8
  sTmDiag_D_u8HiSidePFltSt : Inport  Port=2  OutDataTypeStr=uint8
  sTmDiag_D_u8OutrCondOutTFltSt : Inport  Port=3  OutDataTypeStr=uint8
  sTmIn_D_u8HeatPump : Inport  Port=4  OutDataTypeStr=uint8
  sTmDiag_D_u8HiSidePNHPFltSt : Inport  Port=5  OutDataTypeStr=uint8
  Compare To Constant{,1..2,6} (4 alike) : simulink/Logic and Bit Operations/Compare To Constant  relop=~=  const=0  OutDataTypeStr=boolean
  Compare To Constant3 : simulink/Logic and Bit Operations/Compare To Constant  relop===  const=2  OutDataTypeStr=boolean
  Compare To Constant4 : simulink/Logic and Bit Operations/Compare To Constant  relop===  const=2  OutDataTypeStr=boolean
  Compare To Constant5 : simulink/Logic and Bit Operations/Compare To Constant  relop===  const=2  OutDataTypeStr=boolean
  Compare To Constant7 : simulink/Logic and Bit Operations/Compare To Constant  relop===  const=1  OutDataTypeStr=boolean
  Constant : Constant  Value=cTmComprCtrl_n_u16CmpMaxSpdSensorFltLimt  OutDataTypeStr=uint16
  Constant1 : Constant  Value=8000  OutDataTypeStr=uint16
  Logical Operator : Logic  Operator=OR  Inputs=4  AllPortsSameDT=off  OutDataTypeStr=boolean
  Logical Operator{1..4} (4 alike) : Logic  AllPortsSameDT=off  OutDataTypeStr=boolean
  Switch : Switch  Criteria=u2 ~= 0  SaturateOnIntegerOverflow=off  InputSameDT=off
  rTmComprCtrl_n_u16CompMaxRpmSensFlt : Outport  OutDataTypeStr=uint16
  xTmComprCtrl_B_CmpSensorFltLimtFlag : Outport  Port=2  OutDataTypeStr=boolean
  wires:
  [sTmDiag_D_u8HiSidePFltSt] -> Compare To Constant/1
  [sTmDiag_D_u8OutrCondOutTFltSt] -> Compare To Constant1/1
  [sTmDiag_D_u8CmprDischrgTFltSt] -> Compare To Constant2/1
  Constant/1 -> Switch/1
  Switch/1 -> [rTmComprCtrl_n_u16CompMaxRpmSensFlt]  "rTmComprCtrl_n_u16CompMaxRpmSensFlt"
  Constant1/1 -> Switch/3
  sTmDiag_D_u8CmprDischrgTFltSt/1 -> [sTmDiag_D_u8CmprDischrgTFltSt]  "sTmDiag_D_u8CmprDischrgTFltSt"
  sTmDiag_D_u8HiSidePFltSt/1 -> [sTmDiag_D_u8HiSidePFltSt]  "sTmDiag_D_u8HiSidePFltSt"
  sTmDiag_D_u8OutrCondOutTFltSt/1 -> [sTmDiag_D_u8OutrCondOutTFltSt]  "sTmDiag_D_u8OutrCondOutTFltSt"
  [rTmComprCtrl_n_u16CompMaxRpmSensFlt] -> rTmComprCtrl_n_u16CompMaxRpmSensFlt/1  "rTmComprCtrl_n_u16CompMaxRpmSensFlt"
  Logical Operator/1 -> [xTmComprCtrl_B_CmpSensorFltLimtFlag]
  [xTmComprCtrl_B_CmpSensorFltLimtFlag] -> xTmComprCtrl_B_CmpSensorFltLimtFlag/1  "xTmComprCtrl_B_CmpSensorFltLimtFlag"
  [xTmComprCtrl_B_CmpSensorFltLimtFlag] -> Switch/2
  [sTmIn_D_u8HeatPump] -> Compare To Constant3/1
  Compare To Constant3/1 -> Logical Operator1/1
  Compare To Constant1/1 -> Logical Operator1/2
  [sTmIn_D_u8HeatPump] -> Compare To Constant4/1
  Compare To Constant4/1 -> Logical Operator2/1
  Compare To Constant2/1 -> Logical Operator2/2
  sTmIn_D_u8HeatPump/1 -> [sTmIn_D_u8HeatPump]  "sTmIn_D_u8HeatPump"
  [sTmIn_D_u8HeatPump] -> Compare To Constant5/1
  Compare To Constant/1 -> Logical Operator3/2
  Compare To Constant5/1 -> Logical Operator3/1
  Compare To Constant6/1 -> Logical Operator4/2
  [sTmIn_D_u8HeatPump] -> Compare To Constant7/1
  [sTmDiag_D_u8HiSidePNHPFltSt] -> Compare To Constant6/1
  Compare To Constant7/1 -> Logical Operator4/1
  Logical Operator1/1 -> Logical Operator/3
  Logical Operator2/1 -> Logical Operator/4
  Logical Operator3/1 -> Logical Operator/2
  Logical Operator4/1 -> Logical Operator/1
  sTmDiag_D_u8HiSidePNHPFltSt/1 -> [sTmDiag_D_u8HiSidePNHPFltSt]  "sTmDiag_D_u8HiSidePNHPFltSt"

== system ScriptDemo/Create/Model/createModGotoAll/After/TAmbLimit ==
  note: 0703：
      | 新增 rTmComprCtrl_n_u16CompMaxRpmTAmb 标定开关，可以通过强标成8000，来屏蔽NVH限制
  sTmSigProces_Pw_i16ReqPwrForHeat : Inport  OutDataTypeStr=int16
  rTmComprCtrl_n_u16CompRpmReqBoundary : Inport  Port=2  OutDataTypeStr=uint16
  Compare To Constant : simulink/Logic and Bit Operations/Compare To Constant  relop===  const=[4 5 6]  OutDataTypeStr=boolean
  Logical Operator : Logic  Operator=NOT  AllPortsSameDT=off  OutDataTypeStr=boolean
  Logical Operator1 : Logic  Operator=OR  Inputs=1  AllPortsSameDT=off  OutDataTypeStr=boolean
  Merge : Merge
  Merge1 : Merge
  OutDebugRvs : PCMULib/Interface/OutdebugRvs  SWI=cTmComprCtrl_n_u16CompMaxRpmTAmb_sw  DBI=cTmComprCtrl_n_u16CompMaxRpmTAmb_db
      settings: SourceProductName=PCMULib
  SM456 : Subsystem  TreatAsAtomicUnit=on
  SM456E : Subsystem  TreatAsAtomicUnit=on
  rTmComprCtrl_n_u16CompMaxRpmTAmb : Outport  OutDataTypeStr=uint16
  xTmComprCtrl_B_CmpAmbLimtFlag : Outport  Port=2  OutDataTypeStr=boolean
  wires:
  sTmSigProces_Pw_i16ReqPwrForHeat/1 -> [sTmSigProces_Pw_i16ReqPwrForHeat]
  ? -> [sTmSigProces_Te_s32TAmb]
  [sTmComprCtrl_n_u16CompMaxRpm] -> OutDebugRvs/1
  [xTmComprCtrl_B_CmpAmbLimtFlag] -> xTmComprCtrl_B_CmpAmbLimtFlag/1
  rTmComprCtrl_n_u16CompRpmReqBoundary/1 -> [rTmComprCtrl_n_u16CompRpmReqBoundary]
  [sTmRefriModeMgr_D_u8HPCurMode] -> Compare To Constant/1
  Compare To Constant/1 -> Logical Operator1/1
  Logical Operator/1 -> SM456E/Enable
  [rTmComprCtrl_n_u16CompRpmReqBoundary] -> SM456/1(rTmComprCtrl_n_u16CompRpmReqBoundary)
  [sTmSigProces_Te_s32TAmb] -> ?
  [sTmSigProces_Pw_i16ReqPwrForHeat] -> SM456/2(sTmSigProces_Pw_i16ReqPwrForHeat)
  SM456/1(xSM456_B_CmpMaxSpdForAmbFlag) -> [xSM456_B_CmpMaxSpdForAmbFlag]
  SM456/2(sSM456_n_u16CompMaxRpm) -> [sSM456_n_u16CompMaxRpm]
  SM456E/1(sSM456E_n_u16CompMaxRpm) -> [sSM456E_n_u16CompMaxRpm]
  SM456E/2(xSM456E_B_CmpMaxSpdForAmbFlag) -> [xSM456E_B_CmpMaxSpdForAmbFlag]
  [xSM456_B_CmpMaxSpdForAmbFlag] -> Merge/1
  [xSM456E_B_CmpMaxSpdForAmbFlag] -> Merge/2
  Merge/1 -> [xTmComprCtrl_B_CmpAmbLimtFlag]
  [sSM456_n_u16CompMaxRpm] -> Merge1/1
  [sSM456E_n_u16CompMaxRpm] -> Merge1/2
  Merge1/1 -> [sTmComprCtrl_n_u16CompMaxRpm]
  ? -> [sTmRefriModeMgr_D_u8HPCurMode]
  Logical Operator1/1 -> Logical Operator/1, SM456/Enable
  OutDebugRvs/1 -> rTmComprCtrl_n_u16CompMaxRpmTAmb/1  "rTmComprCtrl_n_u16CompMaxRpmTAmb"

== system ScriptDemo/Create/Model/createModGotoAll/Before/AFFaultLimit ==
  sTmDiag_D_u8FanFltSt : Inport  OutDataTypeStr=uint8
  Compare To Constant : simulink/Logic and Bit Operations/Compare To Constant  relop=~=  const=0  OutDataTypeStr=boolean
  Constant : Constant  Value=cTmComprCtrl_n_u16CmpMaxSpdFanFltLimt  OutDataTypeStr=uint16
  Constant1 : Constant  Value=8000  OutDataTypeStr=uint16
  Switch : Switch  Criteria=u2 ~= 0  SaturateOnIntegerOverflow=off  InputSameDT=off
  rTmComprCtrl_n_u16CompMaxRpmAfFlt : Outport  OutDataTypeStr=uint16
  xTmComprCtrl_B_CmpFanFltLimtFlag : Outport  Port=2  OutDataTypeStr=boolean
  wires:
  Constant/1 -> Switch/1
  Constant1/1 -> Switch/3
  Switch/1 -> [rTmComprCtrl_n_u16CompMaxRpmAfFlt]  "rTmComprCtrl_n_u16CompMaxRpmAfFlt"
  sTmDiag_D_u8FanFltSt/1 -> [sTmDiag_D_u8FanFltSt]
  [rTmComprCtrl_n_u16CompMaxRpmAfFlt] -> rTmComprCtrl_n_u16CompMaxRpmAfFlt/1
  [sTmDiag_D_u8FanFltSt] -> Compare To Constant/1
  Compare To Constant/1 -> [xTmComprCtrl_B_CmpFanFltLimtFlag]
  [xTmComprCtrl_B_CmpFanFltLimtFlag] -> xTmComprCtrl_B_CmpFanFltLimtFlag/1
  [xTmComprCtrl_B_CmpFanFltLimtFlag] -> Switch/2

== system ScriptDemo/Create/Model/createModGotoAll/Before/LoSidePFltLimt ==
  sTmDiag_D_u8LoSidePFltSt : Inport  OutDataTypeStr=uint8
  sTmIn_D_u8HeatPump : Inport  Port=2  OutDataTypeStr=uint8
  Compare To Constant : simulink/Logic and Bit Operations/Compare To Constant  relop=~=  const=0  OutDataTypeStr=boolean
  Compare To Constant1 : simulink/Logic and Bit Operations/Compare To Constant  relop=>  const=30  OutDataTypeStr=boolean
  Compare To Constant4 : simulink/Logic and Bit Operations/Compare To Constant  relop===  const=2  OutDataTypeStr=boolean
  Constant : Constant  Value=cTmComprCtrl_n_u16CmpMaxSpdLoSidePFltLimt  OutDataTypeStr=uint16
  Constant1 : Constant  Value=8000  OutDataTypeStr=uint16
  Logical Operator : Logic  Inputs=3  AllPortsSameDT=off  OutDataTypeStr=boolean
  Switch : Switch  Criteria=u2 ~= 0  SaturateOnIntegerOverflow=off  InputSameDT=off
  rTmComprCtrl_n_u16CompMaxRpmLoSidePFlt : Outport  OutDataTypeStr=uint16
  xTmComprCtrl_B_CmpLoSidePFltLimtFlag : Outport  Port=2  OutDataTypeStr=boolean
  wires:
  [xTmComprCtrl_B_CmpLoSidePFltLimtFlag] -> Switch/2
  [sTmSigProces_Te_s32TAmb] -> Compare To Constant1/1
  Constant/1 -> Switch/1
  Logical Operator/1 -> [xTmComprCtrl_B_CmpLoSidePFltLimtFlag]
  Switch/1 -> [rTmComprCtrl_n_u16CompMaxRpmLoSidePFlt]  "rTmComprCtrl_n_u16CompMaxRpmLoSidePFlt"
  [sTmDiag_D_u8LoSidePFltSt] -> Compare To Constant/1
  Constant1/1 -> Switch/3
  sTmDiag_D_u8LoSidePFltSt/1 -> [sTmDiag_D_u8LoSidePFltSt]
  ? -> [sTmSigProces_Te_s32TAmb]
  [rTmComprCtrl_n_u16CompMaxRpmLoSidePFlt] -> rTmComprCtrl_n_u16CompMaxRpmLoSidePFlt/1
  [xTmComprCtrl_B_CmpLoSidePFltLimtFlag] -> xTmComprCtrl_B_CmpLoSidePFltLimtFlag/1
  [sTmIn_D_u8HeatPump] -> Compare To Constant4/1
  Compare To Constant/1 -> Logical Operator/2
  Compare To Constant1/1 -> Logical Operator/3
  Compare To Constant4/1 -> Logical Operator/1
  sTmIn_D_u8HeatPump/1 -> [sTmIn_D_u8HeatPump]

== system ScriptDemo/Create/Model/createModGotoAll/Before/SensFaultLimit ==
  sTmDiag_D_u8CmprDischrgTFltSt : Inport  OutDataTypeStr=uint8
  sTmDiag_D_u8HiSidePFltSt : Inport  Port=2  OutDataTypeStr=uint8
  sTmDiag_D_u8OutrCondOutTFltSt : Inport  Port=3  OutDataTypeStr=uint8
  sTmIn_D_u8HeatPump : Inport  Port=4  OutDataTypeStr=uint8
  sTmDiag_D_u8HiSidePNHPFltSt : Inport  Port=5  OutDataTypeStr=uint8
  Compare To Constant{,1..2,6} (4 alike) : simulink/Logic and Bit Operations/Compare To Constant  relop=~=  const=0  OutDataTypeStr=boolean
  Compare To Constant3 : simulink/Logic and Bit Operations/Compare To Constant  relop===  const=2  OutDataTypeStr=boolean
  Compare To Constant4 : simulink/Logic and Bit Operations/Compare To Constant  relop===  const=2  OutDataTypeStr=boolean
  Compare To Constant5 : simulink/Logic and Bit Operations/Compare To Constant  relop===  const=2  OutDataTypeStr=boolean
  Compare To Constant7 : simulink/Logic and Bit Operations/Compare To Constant  relop===  const=1  OutDataTypeStr=boolean
  Constant : Constant  Value=cTmComprCtrl_n_u16CmpMaxSpdSensorFltLimt  OutDataTypeStr=uint16
  Constant1 : Constant  Value=8000  OutDataTypeStr=uint16
  Logical Operator : Logic  Operator=OR  Inputs=4  AllPortsSameDT=off  OutDataTypeStr=boolean
  Logical Operator{1..4} (4 alike) : Logic  AllPortsSameDT=off  OutDataTypeStr=boolean
  Switch : Switch  Criteria=u2 ~= 0  SaturateOnIntegerOverflow=off  InputSameDT=off
  rTmComprCtrl_n_u16CompMaxRpmSensFlt : Outport  OutDataTypeStr=uint16
  xTmComprCtrl_B_CmpSensorFltLimtFlag : Outport  Port=2  OutDataTypeStr=boolean
  wires:
  [sTmDiag_D_u8HiSidePFltSt] -> Compare To Constant/1
  [sTmDiag_D_u8OutrCondOutTFltSt] -> Compare To Constant1/1
  [sTmDiag_D_u8CmprDischrgTFltSt] -> Compare To Constant2/1
  Constant/1 -> Switch/1
  Switch/1 -> [rTmComprCtrl_n_u16CompMaxRpmSensFlt]  "rTmComprCtrl_n_u16CompMaxRpmSensFlt"
  Constant1/1 -> Switch/3
  sTmDiag_D_u8CmprDischrgTFltSt/1 -> [sTmDiag_D_u8CmprDischrgTFltSt]  "sTmDiag_D_u8CmprDischrgTFltSt"
  sTmDiag_D_u8HiSidePFltSt/1 -> [sTmDiag_D_u8HiSidePFltSt]  "sTmDiag_D_u8HiSidePFltSt"
  sTmDiag_D_u8OutrCondOutTFltSt/1 -> [sTmDiag_D_u8OutrCondOutTFltSt]  "sTmDiag_D_u8OutrCondOutTFltSt"
  [rTmComprCtrl_n_u16CompMaxRpmSensFlt] -> rTmComprCtrl_n_u16CompMaxRpmSensFlt/1  "rTmComprCtrl_n_u16CompMaxRpmSensFlt"
  Logical Operator/1 -> [xTmComprCtrl_B_CmpSensorFltLimtFlag]
  [xTmComprCtrl_B_CmpSensorFltLimtFlag] -> xTmComprCtrl_B_CmpSensorFltLimtFlag/1  "xTmComprCtrl_B_CmpSensorFltLimtFlag"
  [xTmComprCtrl_B_CmpSensorFltLimtFlag] -> Switch/2
  [sTmIn_D_u8HeatPump] -> Compare To Constant3/1
  Compare To Constant3/1 -> Logical Operator1/1
  Compare To Constant1/1 -> Logical Operator1/2
  [sTmIn_D_u8HeatPump] -> Compare To Constant4/1
  Compare To Constant4/1 -> Logical Operator2/1
  Compare To Constant2/1 -> Logical Operator2/2
  sTmIn_D_u8HeatPump/1 -> [sTmIn_D_u8HeatPump]  "sTmIn_D_u8HeatPump"
  [sTmIn_D_u8HeatPump] -> Compare To Constant5/1
  Compare To Constant/1 -> Logical Operator3/2
  Compare To Constant5/1 -> Logical Operator3/1
  Compare To Constant6/1 -> Logical Operator4/2
  [sTmIn_D_u8HeatPump] -> Compare To Constant7/1
  [sTmDiag_D_u8HiSidePNHPFltSt] -> Compare To Constant6/1
  Compare To Constant7/1 -> Logical Operator4/1
  Logical Operator1/1 -> Logical Operator/3
  Logical Operator2/1 -> Logical Operator/4
  Logical Operator3/1 -> Logical Operator/2
  Logical Operator4/1 -> Logical Operator/1
  sTmDiag_D_u8HiSidePNHPFltSt/1 -> [sTmDiag_D_u8HiSidePNHPFltSt]  "sTmDiag_D_u8HiSidePNHPFltSt"
